simulink model "sampleModel1554"  (R2023a)
settings: Solver=VariableStepAuto  StartTime=0.0  StopTime=10.0  RelTol=1e-3
libraries: hdlsllib x4, simulink x1
settings Model: Creator=user1  LastModifiedBy=user1

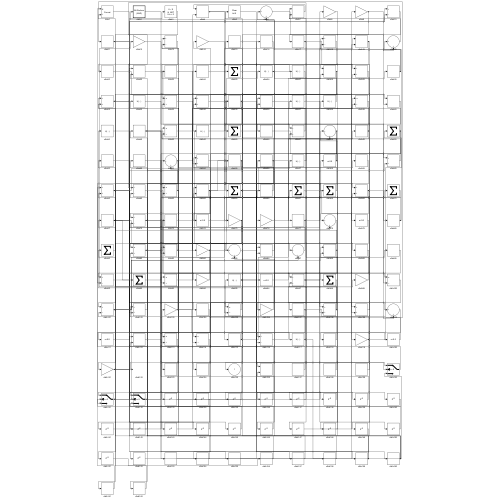
[thumbnail: Simulink's stored preview of the top-level diagram]
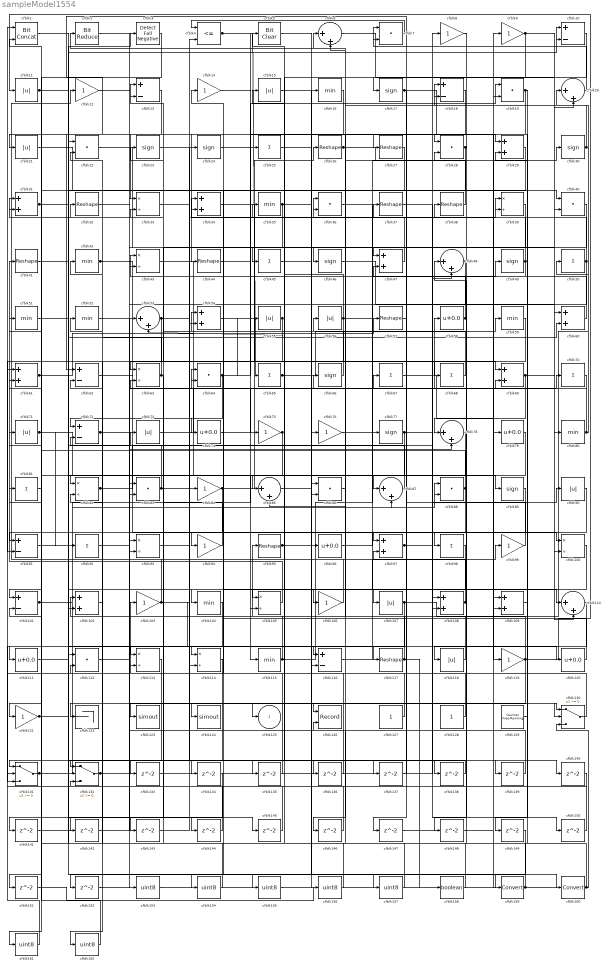
== system sampleModel1554 ==
  cfblk1 : hdlsllib/Logic and Bit Operations/Bit Concat  numInputs=2
  cfblk{10,13,18,62,72,91,101,116} (8 alike) : Sum  Inputs=+-
  cfblk{33,39,43,63,82,93,100,105,113..114} (10 alike) : Product  Inputs=*/  RndMeth=Zero  SaturateOnIntegerOverflow=on
  cfblk{29,31,34,47,54,60..61,69,97,102,108..109} (12 alike) : Sum
  cfblk{8..9,12,14,75..76,84,94,99,103,106,119,121} (13 alike) : Gain
  cfblk{16,35,42,51..52,59,80,104,115} (9 alike) : MinMax
  cfblk{11,15,21,55..56,71,73,90,107,118} (10 alike) : Abs  SaturateOnIntegerOverflow=off
  cfblk{6,20,48,53,78,85,87,110} (8 alike) : Sum  Inputs=|++
  cfblk{58,74,79,96,111,120} (6 alike) : Bias  Bias=0.0  SaturateOnIntegerOverflow=off
  cfblk{7,19,22,28,36,40,64,83,86,88,112} (11 alike) : DotProduct  OutDataTypeStr=Inherit: Inherit via internal rule
  cfblk{26..27,32,37..38,41,44,57,95,117} (10 alike) : Reshape
  cfblk122 : Terminator
  cfblk123 : ToWorkspace  VariableName=simout  SaveFormat=Timeseries  SampleTime=-1
  cfblk124 : ToWorkspace  VariableName=simout  SaveFormat=Timeseries  SampleTime=-1
  cfblk126 : Record  FileSettingsInternal="{\"entries\":[{\"content\":{\"excelSettings\":{\"content\":{},\"type\":\"Streamout.ExcelSettings\"}},\"type\":\"Streamout.FileSettingStorage\",\"uuid\":\"\"}],\"packageUris\":[\"http:\\/\\/schema.mathworks.com\\/mf0\\/streamout_blocks\\/R2020a\"],\"version\":\"1.0\"}"  Layout=[1 1]  SignalsInternal="{\"entries\":[{\"content\":{\"signals\":[{\"content\":{\"blockPath\":[],\"dimensions\":[1],\"domain\":\"\",\"lineColor\":\"#a2142f\",\"plots\":[1],\"port\":1,\"signalID\":1674,\"signalName\":\"XY Graph:1\"},\"type\":\"RecordBlkView.Signal\",\"uuid\":\"\"},{\"content\":{\"blockPath\":[],\"dimensions\":[1],\"domain\":\"\",\"lineColor\":\"#139fff\",\"plots\":[1],\"port\":2,\"signalID\":1677,\"signalName\":\"XY Graph:2\"},\"type\":\"RecordBlkView.Signal\",\"uuid\":\"\"}]},\"type\":\"RecordBlkView.InputSignals\",\"uuid\":\"\"}],\"packageUris\":[\"http:\\/\\/schema.mathworks.com\\/mf0\\/streamout_blocks\\/R2020a\"],\"version\":\"1.0\"}"  VisualizationBindings="{\"xyplotplugin\":{\"info\":[{\"series\":[{\"bindingParametersList\":[{\"parameter\":\"X-Axis\",\"signalID\":1674,\"signalName\":\"XY Graph:1\"},{\"parameter\":\"Y-Axis\",\"signalID\":1677,\"signalName\":\"XY Graph:2\"}],\"seriesID\":22489}],\"subplotID\":1}]}}"  CompatibilityTag=XY  st=-1
  cfblk127 : Constant  SampleTime=-1
  cfblk128 : Constant  SampleTime=-1
  cfblk129 : hdlsllib/Sources/Counter Free-Running  NumBits=16  tsamp=-1
  cfblk130 : Switch  SaturateOnIntegerOverflow=off  InputSameDT=off
  cfblk131 : Switch  SaturateOnIntegerOverflow=off  InputSameDT=off
  cfblk132 : Switch  SaturateOnIntegerOverflow=off  InputSameDT=off
  cfblk{133..152} (20 alike) : Delay  SampleTime=1
  cfblk{153..157,161..162} (7 alike) : DataTypeConversion  OutDataTypeStr=uint8  SaturateOnIntegerOverflow=off  RndMeth=Floor
  cfblk158 : DataTypeConversion  OutDataTypeStr=boolean  SaturateOnIntegerOverflow=off  RndMeth=Floor
  cfblk159 : DataTypeConversion  SaturateOnIntegerOverflow=off  RndMeth=Floor
  cfblk160 : DataTypeConversion  SaturateOnIntegerOverflow=off  RndMeth=Floor
  cfblk{17,23..24,30,46,49,66,77,89} (9 alike) : Signum
  cfblk2 : hdlsllib/Logic and Bit Operations/Bit Reduce  mode=AND
  cfblk{25,45,50,65,67..68,70,81,92,98} (10 alike) : Sum  Inputs=+
  cfblk3 : hdlsllib/Logic and Bit Operations/Detect Fall Negative  vinit=0  OutDataTypeStr=boolean
  cfblk4 : RelationalOperator  Operator=<=  OutDataTypeStr=boolean  InputSameDT=off
  cfblk5 : simulink/Logic and Bit Operations/Bit Clear  iBit=0
      settings: LibrarySourceBlock=|
      | hdlsllib/Logic and Bit
      | Operations/Bit Clear
  cfblk125 : Outport  VectorParamsAs1DForOutWhenUnconnected=off
  wires:
  cfblk84/1 -> cfblk26/1, cfblk102/2
  cfblk39/1 -> cfblk46/1
  cfblk61/1 -> cfblk57/1, cfblk114/2, cfblk105/2
  cfblk130/1 -> cfblk103/1
  cfblk131/1 -> cfblk104/1, cfblk60/2
  cfblk38/1 -> cfblk2/1
  cfblk43/1 -> cfblk85/1
  cfblk106/1 -> cfblk12/1
  cfblk109/1 -> cfblk28/1
  cfblk19/1 -> cfblk44/1, cfblk149/1
  cfblk7/1 -> cfblk4/1
  cfblk60/1 -> cfblk43/1
  cfblk22/1 -> cfblk84/1
  cfblk105/1 -> cfblk41/1
  cfblk75/1 -> cfblk131/1, cfblk143/1
  cfblk4/1 -> cfblk65/1, cfblk27/1
  cfblk108/1 -> cfblk85/2, cfblk81/1
  cfblk88/1 -> cfblk91/1, cfblk61/2
  cfblk103/1 -> cfblk117/1, cfblk71/1, cfblk67/1
  cfblk64/1 -> cfblk72/1, cfblk55/1, cfblk18/2, cfblk124/1
  cfblk20/1 -> cfblk62/1
  cfblk56/1 -> cfblk101/1, cfblk109/2, cfblk35/1, cfblk116/2
  cfblk25/1 -> cfblk76/1
  cfblk42/1 -> cfblk94/1, cfblk68/1, cfblk130/1
  cfblk72/1 -> cfblk97/1, cfblk140/1
  cfblk99/1 -> cfblk37/1
  cfblk93/1 -> cfblk39/1
  cfblk107/1 -> cfblk20/1, cfblk131/3
  cfblk36/1 -> cfblk77/1
  cfblk45/1 -> cfblk69/1
  cfblk26/1 -> cfblk28/2, cfblk146/1
  cfblk17/1 -> cfblk107/1, cfblk109/1
  cfblk47/1 -> cfblk34/1
  cfblk87/1 -> cfblk42/1
  cfblk62/1 -> cfblk87/1
  cfblk13/1 -> cfblk21/1
  cfblk113/1 -> cfblk132/1
  cfblk73/1 -> cfblk70/1
  cfblk79/1 -> cfblk82/1
  cfblk127/1 -> cfblk54/1
  cfblk40/1 -> cfblk45/1
  cfblk116/1 -> cfblk99/1
  cfblk74/1 -> cfblk58/1
  cfblk94/1 -> cfblk13/1
  cfblk65/1 -> cfblk59/1, cfblk157/1
  cfblk53/1 -> cfblk122/1, cfblk36/1
  cfblk66/1 -> cfblk15/1
  cfblk118/1 -> cfblk95/1
  cfblk115/1 -> cfblk30/1, cfblk23/1
  cfblk119/1 -> cfblk11/1, cfblk102/1, cfblk152/1
  cfblk49/1 -> cfblk38/1, cfblk47/2
  cfblk1/1 -> cfblk160/1
  cfblk8/1 -> cfblk98/1
  cfblk59/1 -> cfblk91/2
  cfblk86/1 -> cfblk56/1
  cfblk69/1 -> cfblk78/1, cfblk110/2
  cfblk121/1 -> cfblk10/1, cfblk144/1, cfblk145/1
  cfblk9/1 -> cfblk17/1, cfblk20/2
  cfblk41/1 -> cfblk110/1
  cfblk44/1 -> cfblk25/1
  cfblk67/1 -> cfblk119/1
  cfblk16/1 -> cfblk33/1
  cfblk24/1 -> cfblk29/1
  cfblk28/1 -> cfblk105/1, cfblk121/1
  cfblk111/1 -> cfblk73/1
  cfblk97/1 -> cfblk108/1, cfblk90/1
  cfblk132/1 -> cfblk93/1, cfblk48/2
  cfblk63/1 -> cfblk113/1, cfblk22/2
  cfblk14/1 -> cfblk75/1
  cfblk101/1 -> cfblk88/1, cfblk66/1, cfblk87/2
  cfblk110/1 -> cfblk118/1
  cfblk120/1 -> cfblk34/2
  cfblk76/1 -> cfblk49/1
  cfblk90/1 -> cfblk123/1
  cfblk5/1 -> cfblk159/1
  cfblk77/1 -> cfblk8/1, cfblk106/1
  cfblk55/1 -> cfblk53/2, cfblk142/1
  cfblk117/1 -> cfblk36/2, cfblk158/1
  cfblk18/1 -> cfblk126/1
  cfblk21/1 -> cfblk79/1
  cfblk58/1 -> cfblk6/1, cfblk43/2
  cfblk71/1 -> cfblk115/1, cfblk10/2, cfblk116/1, cfblk92/1
  cfblk57/1 -> cfblk7/1
  cfblk83/1 -> cfblk24/1, cfblk72/2
  cfblk54/1 -> cfblk108/2
  cfblk6/1 -> cfblk60/1
  cfblk35/1 -> cfblk63/1, cfblk130/2
  cfblk10/1 -> cfblk125/1
  cfblk95/1 -> cfblk16/1, cfblk139/1
  cfblk98/1 -> cfblk114/1
  cfblk50/1 -> cfblk14/1, cfblk147/1, cfblk148/1
  cfblk128/1 -> cfblk7/2
  cfblk30/1 -> cfblk18/1, cfblk6/2
  cfblk23/1 -> cfblk54/2
  cfblk52/1 -> cfblk93/2
  cfblk102/1 -> cfblk52/1
  cfblk129/1 -> cfblk29/2
  cfblk15/1 -> cfblk120/1
  cfblk96/1 -> cfblk100/1
  cfblk85/1 -> cfblk39/2
  cfblk104/1 -> cfblk111/1
  cfblk92/1 -> cfblk64/1
  cfblk12/1 -> cfblk78/2
  cfblk81/1 -> cfblk31/1
  cfblk68/1 -> cfblk31/2
  cfblk48/1 -> cfblk74/1, cfblk83/2
  cfblk82/1 -> cfblk113/2, cfblk19/1
  cfblk70/1 -> cfblk63/2
  cfblk51/1 -> cfblk86/2
  cfblk31/1 -> cfblk89/1, cfblk40/1
  cfblk34/1 -> cfblk80/1
  cfblk80/1 -> cfblk64/2, cfblk50/1
  cfblk11/1 -> cfblk3/1, cfblk40/2
  cfblk2/1 -> cfblk47/1
  cfblk46/1 -> cfblk100/2
  cfblk91/1 -> cfblk133/1
  cfblk133/1 -> cfblk86/1
  cfblk100/1 -> cfblk134/1
  cfblk29/1 -> cfblk135/1
  cfblk135/1 -> cfblk101/2
  cfblk89/1 -> cfblk136/1
  cfblk136/1 -> cfblk61/1
  cfblk78/1 -> cfblk137/1
  cfblk137/1 -> cfblk97/2
  cfblk33/1 -> cfblk138/1
  cfblk138/1 -> cfblk132/2
  cfblk139/1 -> cfblk83/1
  cfblk140/1 -> cfblk132/3
  cfblk114/1 -> cfblk141/1
  cfblk141/1 -> cfblk53/1
  cfblk142/1 -> cfblk82/2
  cfblk143/1 -> cfblk4/2
  cfblk144/1 -> cfblk13/2
  cfblk145/1 -> cfblk131/2
  cfblk146/1 -> cfblk22/1
  cfblk147/1 -> cfblk19/2
  cfblk148/1 -> cfblk88/2
  cfblk37/1 -> cfblk150/1
  cfblk150/1 -> cfblk62/2
  cfblk3/1 -> cfblk151/1
  cfblk152/1 -> cfblk130/3
  cfblk32/1 -> cfblk153/1
  cfblk153/1 -> cfblk96/1
  cfblk27/1 -> cfblk154/1
  cfblk154/1 -> cfblk32/1
  cfblk112/1 -> cfblk155/1
  cfblk155/1 -> cfblk9/1
  cfblk151/1 -> cfblk156/1
  cfblk156/1 -> cfblk112/1
  cfblk157/1 -> cfblk112/2
  cfblk158/1 -> cfblk5/1
  cfblk159/1 -> cfblk126/2, cfblk33/2
  cfblk160/1 -> cfblk48/1, cfblk69/2, cfblk51/1
  cfblk134/1 -> cfblk161/1
  cfblk161/1 -> cfblk1/1
  cfblk149/1 -> cfblk162/1
  cfblk162/1 -> cfblk1/2
